simulink model "Ex3"  (R2023a)
settings: Solver=VariableStepAuto  StartTime=0.0  StopTime=10.0  RelTol=1e-3
libraries: simulink x1
settings Model: Creator=Aman  LastModifiedBy=Aman

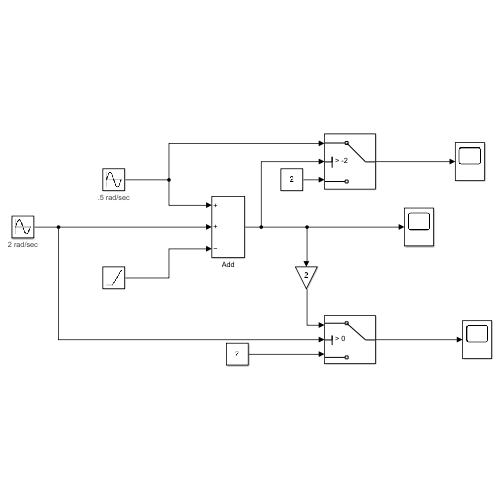
[thumbnail: Simulink's stored preview of the top-level diagram]
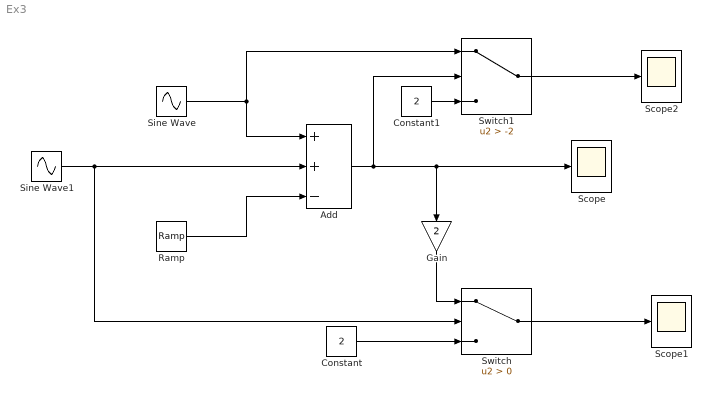
== system Ex3 ==
  Add : Sum  Inputs=++-
  Constant : Constant  Value=2
  Constant1 : Constant  Value=2
  Gain : Gain  Gain=2
  Ramp : simulink/Sources/Ramp  slope=1  start=0  InitialOutput=0
  Scope : Scope
  Scope1 : Scope
  Scope2 : Scope
  Sine Wave : Sin  Frequency=.5  SampleTime=0
      settings: AttributesFormatString=%<Frequency> rad/sec
  Sine Wave1 : Sin  Frequency=2  SampleTime=0
      settings: AttributesFormatString=%<Frequency> rad/sec
  Switch : Switch  Criteria=u2 > Threshold  SaturateOnIntegerOverflow=off  InputSameDT=off
  Switch1 : Switch  Criteria=u2 > Threshold  Threshold=-2  SaturateOnIntegerOverflow=off  InputSameDT=off
  wires:
  Add/1 -> Scope/1, Gain/1, Switch1/2
  Sine Wave1/1 -> Switch/2, Add/2
  Ramp/1 -> Add/3
  Sine Wave/1 -> Switch1/1, Add/1
  Switch/1 -> Scope1/1
  Gain/1 -> Switch/1
  Constant/1 -> Switch/3
  Switch1/1 -> Scope2/1
  Constant1/1 -> Switch1/3
